simulink model "robot"  (R2024a)
settings: Solver=ode4  StartTime=0.0  StopTime=10  FixedStep=5e-5  RelTol=1e-3
settings Model: Creator=pranav  LastModifiedBy=pranav

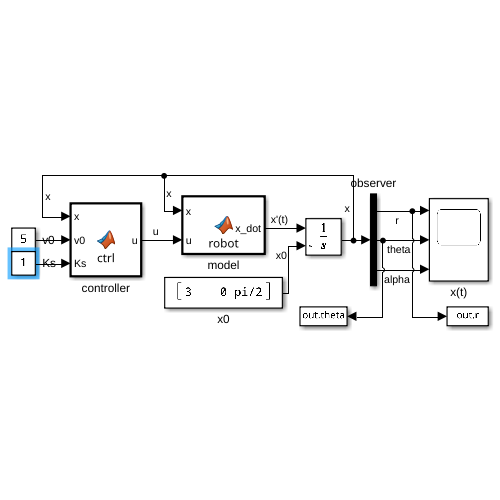
[thumbnail: Simulink's stored preview of the top-level diagram]
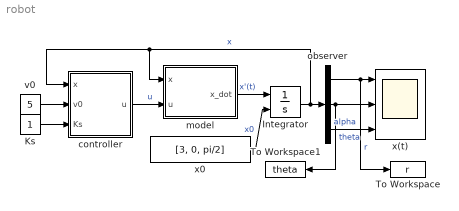
== system robot ==
  Integrator : Integrator  InitialConditionSource=external
  Ks : Constant
  To Workspace : ToWorkspace  VariableName=r  SaveFormat=Timeseries  SampleTime=-1
  To Workspace1 : ToWorkspace  VariableName=theta  SaveFormat=Timeseries  SampleTime=-1
  controller : MATLAB Function  TreatAsAtomicUnit=on
  model : MATLAB Function  TreatAsAtomicUnit=on
  observer : Demux  Outputs=3
  v0 : Constant  Value=5
  x(t) : Scope  NumInputPorts=3
  x0 : Constant  Value=[3, 0, pi/2]
  wires:
  model/1(x_dot) -> Integrator/1  "x'(t)"
  controller/1(u) -> model/2(u)  "u"
  v0/1 -> controller/2(v0)
  Ks/1 -> controller/3(Ks)
  Integrator/1 -> controller/1(x), model/1(x), observer/1  "x"
  x0/1 -> Integrator/2  "x0"
  observer/2 -> x(t)/2, To Workspace1/1  "theta"
  observer/1 -> To Workspace/1, x(t)/1  "r"
  observer/3 -> x(t)/3  "alpha"

== matlab function robot/controller ==
  data: x input; v0 input; u output; Ks input
function u = ctrl(x, v0, Ks)
    % seperating states
    r     = x(1);
    theta = x(2);
    alpha = x(3);

    % computing control inputs
    v     = v0; % * (1-exp(-r/r0));
    omega = -Ks * sign(alpha-(theta+pi));

    % consolidating control
    u = [v, omega];

== matlab function robot/model ==
  data: x input; u input; x_dot output
function x_dot = robot(x, u)
    % seperating states
    r     = x(1);
    theta = x(2);
    alpha = x(3);

    % seperating control inputs
    v     = u(1);
    omega = u(2);

    % kinematic model
    r_dot     = v     * cos(alpha-theta);
    theta_dot = (v/r) * sin(alpha-theta);
    alpha_dot = omega;
    
    % consolidating model
    x_dot = [r_dot, theta_dot, alpha_dot];
